simulink model "chap8_7sim"  (R2015a)
settings: Solver=ode45  StartTime=0.0  StopTime=10  RelTol=1e-3
settings Model: Creator=zhr  LastModifiedBy=zhr

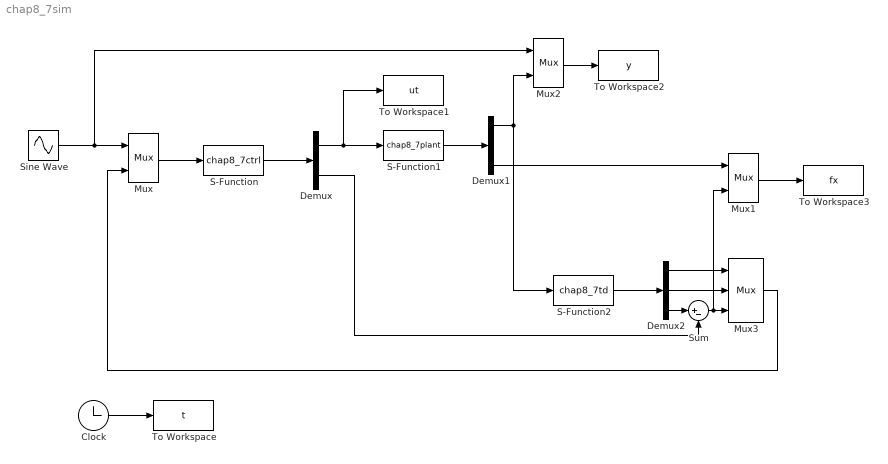
== system chap8_7sim ==
  Clock : Clock
  Demux : Demux  Outputs=2
  Demux1 : Demux  Outputs=3
  Demux2 : Demux  Outputs=3
  Mux : Mux  Inputs=2
  Mux1 : Mux  Inputs=2
  Mux2 : Mux  Inputs=2
  Mux3 : Mux  Inputs=3
  S-Function : S-Function  FunctionName=chap8_7ctrl
  S-Function1 : S-Function  FunctionName=chap8_7plant
  S-Function2 : S-Function  FunctionName=chap8_7td
  Sine Wave : Sin  Amplitude=0.1  SampleTime=0
  Sum : Sum  Inputs=|+-
  To Workspace : ToWorkspace  VariableName=t  SampleTime=-1
  To Workspace1 : ToWorkspace  VariableName=ut  SampleTime=-1
  To Workspace2 : ToWorkspace  VariableName=y  SampleTime=-1
  To Workspace3 : ToWorkspace  VariableName=fx  SampleTime=-1
  wires:
  Clock/1 -> To Workspace/1
  Sine Wave/1 -> Mux2/1, Mux/1
  Mux/1 -> S-Function/1
  S-Function/1 -> Demux/1
  Demux/1 -> To Workspace1/1, S-Function1/1
  S-Function1/1 -> Demux1/1
  Demux1/3 -> Mux1/1
  Demux1/1 -> Mux2/2, S-Function2/1
  S-Function2/1 -> Demux2/1
  Demux2/1 -> Mux3/1
  Demux2/2 -> Mux3/2
  Demux2/3 -> Sum/1
  Sum/1 -> Mux1/2, Mux3/3
  Demux/2 -> Sum/2
  Mux3/1 -> Mux/2
  Mux2/1 -> To Workspace2/1
  Mux1/1 -> To Workspace3/1
